simulink model "PotHoleHDLDetector"  (R2022a)
settings: Solver=FixedStepDiscrete  StartTime=0.0  StopTime=9  RelTol=1e-3
PreLoadFcn:
  | % Straight lines between these corners left,right and top,bottom
  | %        ltc---rtc
  | %        /       \
  | %       /         \
  | %      /           \
  | %   lbc-------------rbc
  | %
  | % For the 320x180 image:
  | raster = [320,180];
  | ltc = [155, 66];
  | lbc = [  1,140];
  | rtc = [155, 66];
  | rbc = [285,179];
  | 
  | % fit to x = f(y) for convienence
  | abl = polyfit([lbc(2),ltc(2)],[lbc(1),ltc(1)],1);  % left side
  | abr = polyfit([rbc(2),rtc(2)],[rbc(1),rtc(1)],1);  % right side
  | leftxstart = max(  1, round((ltc(2):rbc(2))*abl(1)+abl(2)));
  | rightxend  = min(raster(1), round((ltc(2):rbc(2))*abr(1)+abr(2)));
  | startline  = min(ltc(2),rtc(2));
  | endline    = max(lbc(2),rbc(2));
  | % correct values to zero-based
  | leftxstart = leftxstart - 1;
  | rightxend = rightxend - 1;
  | startline = startline - 1;
  | endline = endline - 1;
  | %%%%%%%%%%%%%%%%
  | % Character ROM for OSD
  | load charROM16x16.mat
  | %%%%%%%%%%%%%%%%
  | % Fiducial Marker (square reticle)
  | load fiducialROM31x31.mat
undefined symbols (not defined in the file or in its folder): charROM16x16, fiducialROM, gray, Rec, SDTV
libraries: hdlsllib x62, simulink x18, visionhdlutilities x7, visionhdlio x2, dspvision x1, visionhdlfilter x1, visionhdlmorphops x1, visionhdlconversions x1, visionhdlanalysis x1
(part 2 of 2)

== system PotHoleHDLDetector/PotHoleHDL/Centroid31/CentroidKernel/For Each Subsystem ==
  pixelIn : Inport  Partition=on  PartitionDimension=1  PartitionWidth=1  PartitionOffset=0
  enable : Inport  Port=2
  Delay1 : Delay
  Delay2 : Delay  DelayLength=5
  Delay3 : Delay
  EnTapDelay22 : Subsystem
  For Each : ForEach  DisableCoverage=on
  Gain : Gain  Gain=[-15:15]  ParamDataTypeStr=fixdt(1,5,0)  OutDataTypeStr=fixdt(1,5,0)
  Sum : Sum  Inputs=1
  sumOut : Outport  ConcatenationDimension=1  VectorParamsAs1DForOutWhenUnconnected=off
  wires:
  pixelIn/1 -> EnTapDelay22/1(In1)
  Sum/1 -> Delay2/1
  enable/1 -> EnTapDelay22/Enable
  EnTapDelay22/1(Out1) -> Delay3/1
  Delay3/1 -> Gain/1
  Gain/1 -> Delay1/1
  Delay1/1 -> Sum/1
  Delay2/1 -> sumOut/1

== system PotHoleHDLDetector/PotHoleHDL/Centroid31/CentroidKernel/For Each Subsystem/EnTapDelay22 ==
  In1 : Inport
  Enable : EnablePort
  State Control : StateControl  StateControl=Synchronous
  Tapped Delay : simulink/Discrete/Tapped Delay  vinit=0.0  samptime=-1  NumDelays=31  DelayOrder=Oldest  includeCurrent=off
  Out1 : Outport  VectorParamsAs1DForOutWhenUnconnected=off
  wires:
  In1/1 -> Tapped Delay/1
  Tapped Delay/1 -> Out1/1
